simulink model "microgrid"  (R2025a)
settings: Solver=VariableStepAuto  StartTime=0.0  StopTime=1  RelTol=1e-3
values from neighbouring files (symbols this model uses):
  Cf = 5e-6    (= 5e-06)    [parametros_micro.m]    (also in parametros_micro2.m)
  L = 5e-3    (= 0.005)    [der.m]    (also in der_delay.m; der_delay_mpc.m; der_mpc.m; der_mpc_acoplado.m)
  Lf = 1e-3    (= 0.001)    [parametros_micro.m]    (also in parametros_micro2.m)
  R = 0.1    [der.m]    (also in der_delay.m; der_delay_mpc.m; der_mpc.m; der_mpc_acoplado.m)
libraries: mpclib x1
settings Model: Creator=cmparedesv  LastModifiedBy=cmparedesv

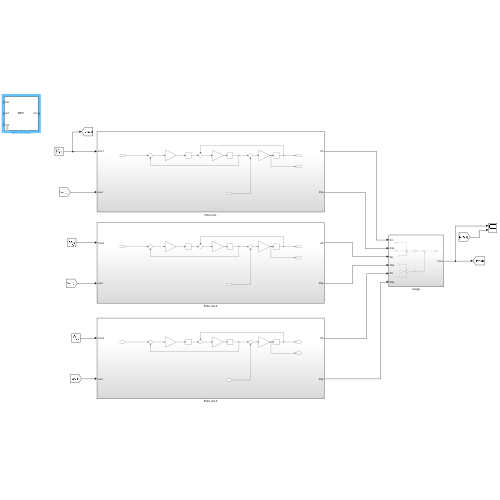
[thumbnail: Simulink's stored preview of the top-level diagram]
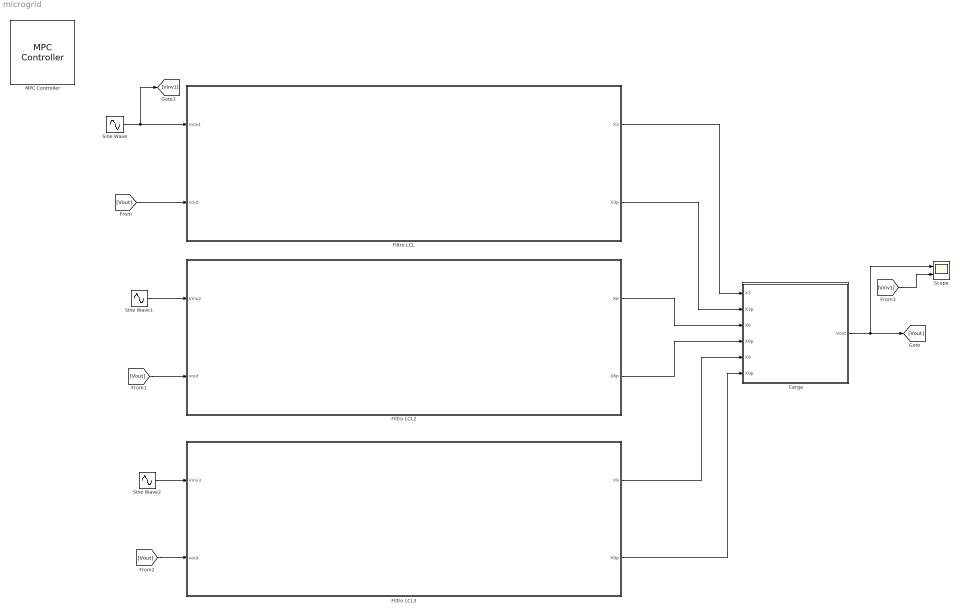
== system microgrid ==
  Carga : Subsystem
  Filtro LCL : Subsystem
  Filtro LCL2 : Subsystem
  Filtro LCL3 : Subsystem
  MPC Controller : mpclib/MPC Controller  SCDEnableBlockLinearizationSpecification=on  is_multiple=0  enable_value=0  return_u0=off  updateMPCinCallerWorkspace=on  md_inport=on  mv_inport=off  uref_inport=off  return_cost=off  return_mvseq=off  return_qpstatus=off  return_xseq=off  return_state=off  return_ovseq=off  state_inport=off  umin_inport=off  umax_inport=off  ymin_inport=off  ymax_inport=off  cc_inport=off  ywt_inport=off  uwt_inport=off  duwt_inport=off  rhoeps_inport=off  pm_inport=off  MaximumP=10  HorizonChoice=FixedHorizon  n_ts=1  n_p=10  n_mv=1  n_md=1  n_ud=0  n_mo=1  n_uo=0  BlockDataType=double  SampleTimeInherited=off  switch_inport=off
  Scope : Scope  NumInputPorts=2
      settings: ActiveDisplayYMinimum=-44.557924874774187  ActiveDisplayYMaximum=213.826682928808
  Sine Wave : Sin  Amplitude=170  Frequency=2*pi*60  SampleTime=0
  Sine Wave1 : Sin  Amplitude=170  Frequency=2*pi*60  SampleTime=0
  Sine Wave2 : Sin  Amplitude=170  Frequency=2*pi*60  SampleTime=0
  wires:
  Filtro LCL/1(X3) -> Carga/1(X3)
  Filtro LCL/2(X3p) -> Carga/2(X3p)
  Filtro LCL2/1(X6) -> Carga/3(X6)
  Filtro LCL2/2(X6p) -> Carga/4(X6p)
  Filtro LCL3/1(X9) -> Carga/5(X9)
  Filtro LCL3/2(X9p) -> Carga/6(X9p)
  Carga/1(Vout) -> Scope/1, [Vout]
  [Vout] -> Filtro LCL/2(vout)
  [Vout] -> Filtro LCL2/2(vout)
  [Vout] -> Filtro LCL3/2(vout)
  Sine Wave/1 -> [Vinv1], Filtro LCL/1(Vinv1)
  Sine Wave1/1 -> Filtro LCL2/1(Vinv2)
  Sine Wave2/1 -> Filtro LCL3/1(Vinv3)
  [Vinv1] -> Scope/2

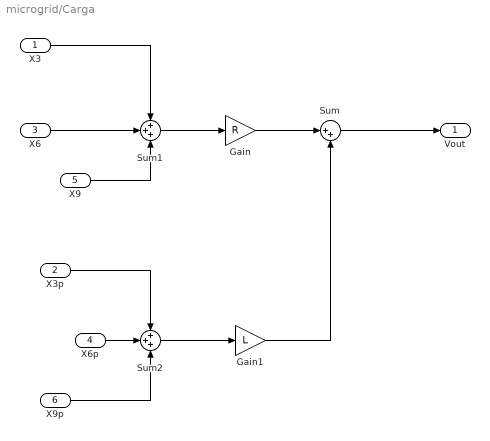
== system microgrid/Carga ==
  X3 : Inport
  X3p : Inport  Port=2
  X6 : Inport  Port=3
  X6p : Inport  Port=4
  X9 : Inport  Port=5
  X9p : Inport  Port=6
  Gain : Gain  Gain=R
  Gain1 : Gain  Gain=L
  Sum : Sum  Inputs=|++
  Sum1 : Sum  Inputs=+++
  Sum2 : Sum  Inputs=+++
  Vout : Outport
  wires:
  Gain/1 -> Sum/1
  Sum2/1 -> Gain1/1
  Gain1/1 -> Sum/2
  Sum/1 -> Vout/1
  Sum1/1 -> Gain/1
  X3/1 -> Sum1/1
  X6/1 -> Sum1/2
  X9/1 -> Sum1/3
  X3p/1 -> Sum2/1
  X6p/1 -> Sum2/2
  X9p/1 -> Sum2/3

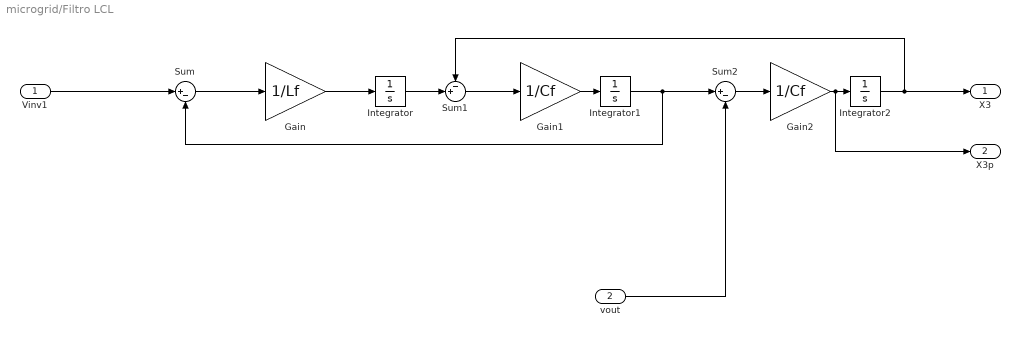
== system microgrid/Filtro LCL ==
  Vinv1 : Inport
  vout : Inport  Port=2
  Gain : Gain  Gain=1/Lf
  Gain1 : Gain  Gain=1/Cf
  Gain2 : Gain  Gain=1/Cf
  Integrator : Integrator
  Integrator1 : Integrator
  Integrator2 : Integrator
  Sum : Sum  Inputs=|+-
  Sum1 : Sum  Inputs=-+|
  Sum2 : Sum  Inputs=|+-
  X3 : Outport
  X3p : Outport  Port=2
  wires:
  Integrator2/1 -> X3/1, Sum1/1
  Integrator/1 -> Sum1/2
  Integrator1/1 -> Sum/2, Sum2/1
  Sum/1 -> Gain/1
  Gain/1 -> Integrator/1
  Sum2/1 -> Gain2/1
  Sum1/1 -> Gain1/1
  Gain1/1 -> Integrator1/1
  Gain2/1 -> X3p/1, Integrator2/1
  vout/1 -> Sum2/2
  Vinv1/1 -> Sum/1

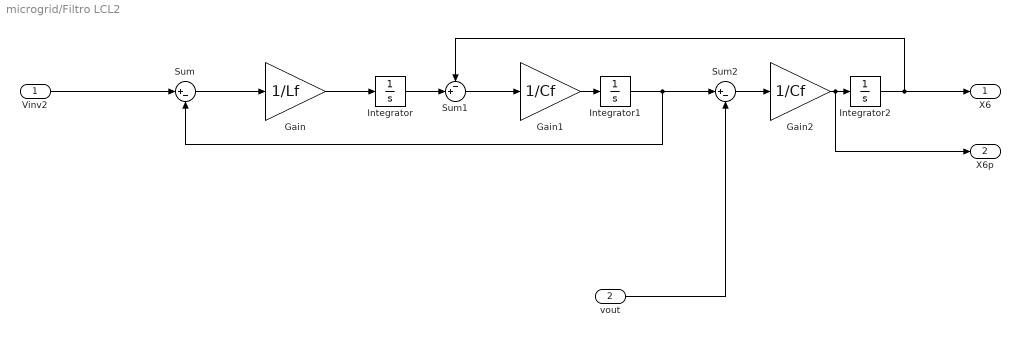
== system microgrid/Filtro LCL2 ==
  Vinv2 : Inport
  vout : Inport  Port=2
  Gain : Gain  Gain=1/Lf
  Gain1 : Gain  Gain=1/Cf
  Gain2 : Gain  Gain=1/Cf
  Integrator : Integrator
  Integrator1 : Integrator
  Integrator2 : Integrator
  Sum : Sum  Inputs=|+-
  Sum1 : Sum  Inputs=-+|
  Sum2 : Sum  Inputs=|+-
  X6 : Outport
  X6p : Outport  Port=2
  wires:
  Integrator2/1 -> X6/1, Sum1/1
  Integrator/1 -> Sum1/2
  Integrator1/1 -> Sum/2, Sum2/1
  Sum/1 -> Gain/1
  Gain/1 -> Integrator/1
  Sum2/1 -> Gain2/1
  Sum1/1 -> Gain1/1
  Gain1/1 -> Integrator1/1
  Gain2/1 -> X6p/1, Integrator2/1
  vout/1 -> Sum2/2
  Vinv2/1 -> Sum/1

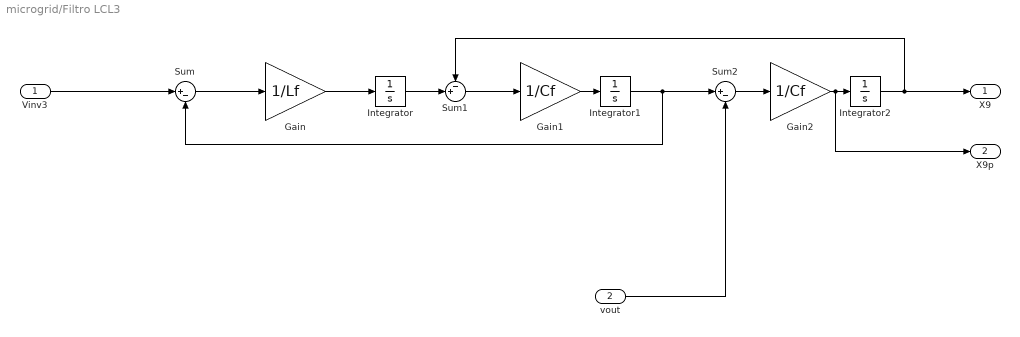
== system microgrid/Filtro LCL3 ==
  Vinv3 : Inport
  vout : Inport  Port=2
  Gain : Gain  Gain=1/Lf
  Gain1 : Gain  Gain=1/Cf
  Gain2 : Gain  Gain=1/Cf
  Integrator : Integrator
  Integrator1 : Integrator
  Integrator2 : Integrator
  Sum : Sum  Inputs=|+-
  Sum1 : Sum  Inputs=-+|
  Sum2 : Sum  Inputs=|+-
  X9 : Outport
  X9p : Outport  Port=2
  wires:
  Integrator2/1 -> X9/1, Sum1/1
  Integrator/1 -> Sum1/2
  Integrator1/1 -> Sum/2, Sum2/1
  Sum/1 -> Gain/1
  Gain/1 -> Integrator/1
  Sum2/1 -> Gain2/1
  Sum1/1 -> Gain1/1
  Gain1/1 -> Integrator1/1
  Gain2/1 -> X9p/1, Integrator2/1
  vout/1 -> Sum2/2
  Vinv3/1 -> Sum/1
